simulink model "ev3_gyroboy_simulink_tcpip"  (R2024a)
settings: Solver=FixedStepDiscrete  StartTime=0.0  StopTime=inf  FixedStep=T_sampling  RelTol=1e-3  EnableMultiTasking=on
undefined symbols (not defined in the file): backward_speed, D_increment, D_max, D_min, DiscIntNeverNeededParam, forward_speed, initial_tilt, k_D_move, k_D_tilt, k_P_move, k_P_tilt, P_increment, P_max, P_min, T_sampling, tilt_limit, turning_speed
libraries: legoev3lib x19, powerlib_meascontrol x2, simulink x1, simulink_extras x1
settings Model: ExtModeTrigDuration=2  Creator=Barteq
settings SolverCC: AlgebraicLoopSolver=TrustRegion  PositivePriorityOrder=on
settings DataIOCC: ReturnWorkspaceOutputs=off
settings OptimizationCC: EnhancedBackFolding=on  PassReuseOutputArgsThreshold=0  MaxStackSize=64  OptimizeBlockOrder=speed  DifferentSizesBufferReuse=on  OptimizationCustomize=off
settings DebuggingCC: ParameterTunabilityLossMsg=error  UnconnectedInputMsg=warning  UnconnectedOutputMsg=warning  UnconnectedLineMsg=warning  ArithmeticOperatorsInVariantConditions=warning
settings HardwareCC: ProdBitPerPointer=32  ProdBitPerSizeT=32  ProdBitPerPtrDiffT=32  ProdLargestAtomicInteger=Long  ProdWordSize=32  ProdHWDeviceType=ARM Compatible->ARM 9
settings ModelReferenceCC: EnableRefExpFcnMdlSchedulingChecks=on
settings SFSimCC: SimUseLocalCustomCode=off  MATLABDynamicMemAlloc=off  CustomCodeUndefinedFunction=UseInterfaceOnly
settings RTWCC: Description=Embedded Coder  SystemTargetFile=ert.tlc  HardwareBoard=LEGO MINDSTORMS EV3  TLCOptions="-aInlineSetEventsForThisBaseRateFcn=TLC_FALSE -aSuppressMultiTaskScheduler=TLC_FALSE  -aRateBasedStepFcn=0"  TemplateMakefile=ert_default_tmf  RTWUseLocalCustomCode=off  Toolchain=Sourcery G++ Lite v2009q3  GPUComputeCapability=3.5
settings CodeAppCC: ForceParamTrailComments=on  OperatorAnnotations=on
settings ERTTargetCC: ERTCustomFileBanners=off  SupportContinuousTime=on  SupportNonInlinedSFcns=on  RemoveResetFunc=off  SupportVariableSizeSignals=on  ModelStepFunctionPrototypeControlCompliant=off
settings ConfigComp: CovBoundaryAbsTol=1.0e-5

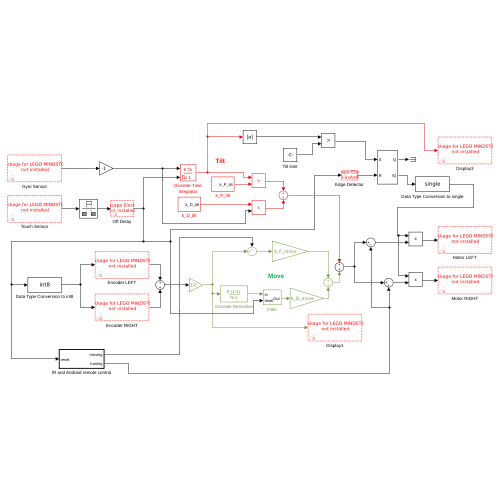
[thumbnail: Simulink's stored preview of the top-level diagram]
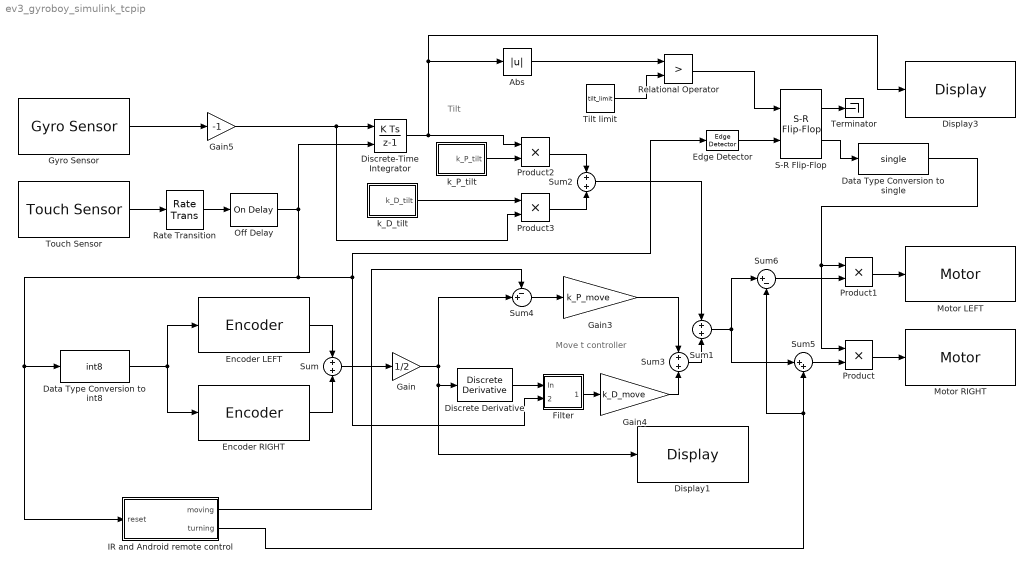
== system ev3_gyroboy_simulink_tcpip ==
  note: Tilt
  note: Move
      | t controller
  Abs : Abs  SaturateOnIntegerOverflow=off
  Data Type Conversion to int8 : DataTypeConversion  OutDataTypeStr=int8  SaturateOnIntegerOverflow=off  RndMeth=Floor
  Data Type Conversion to single : DataTypeConversion  OutDataTypeStr=single  SaturateOnIntegerOverflow=off  RndMeth=Floor
  Discrete Derivative : simulink/Discrete/Discrete Derivative  gainval=1.0  ICPrevScaledInput=0.0  OutMin=[]  OutMax=[]  OutDataTypeStr=single  OutputDataTypeScalingMode=single  OutDataType=fixdt(1, 16)  OutScaling=2^-10  DoSatur=off
  Discrete-Time Integrator : DiscreteIntegrator  ExternalReset=level  InitialCondition=initial_tilt  SampleTime=T_sampling  OutDataTypeStr=single  ICPrevOutput=DiscIntNeverNeededParam  ICPrevScaledInput=DiscIntNeverNeededParam
  Display1 : legoev3lib/Display  slcdStr=Encoders  slcdLine=6  slcdFormat=Decimal
      settings: SourceProductName=Simulink Support Package for LEGO MINDSTORMS EV3 Hardware
  Display3 : legoev3lib/Display  slcdStr=Tilt  slcdLine=4  slcdFormat=Decimal
      settings: SourceProductName=Simulink Support Package for LEGO MINDSTORMS EV3 Hardware
  Edge Detector : powerlib_meascontrol/Logic/Edge Detector  model=Falling  ic=0  Ts=T_sampling
      settings: SourceProductName=Simscape Power Systems
  Encoder LEFT : legoev3lib/Encoder  portNumber=B  opMode=Reset by external signal  sampleTime=T_sampling
      settings: SourceProductName=Simulink Support Package for LEGO MINDSTORMS EV3 Hardware
  Encoder RIGHT : legoev3lib/Encoder  portNumber=D  opMode=Reset by external signal  sampleTime=T_sampling
      settings: SourceProductName=Simulink Support Package for LEGO MINDSTORMS EV3 Hardware
  Filter : Subsystem
  Gain : Gain  Gain=1/2
  Gain3 : Gain  Gain=k_P_move
  Gain4 : Gain  Gain=k_D_move
  Gain5 : Gain  Gain=-1  OutDataTypeStr=single
  Gyro Sensor : legoev3lib/Gyro Sensor  portNumber=2  sampleTime=T_sampling
      settings: SourceProductName=Simulink Support Package for LEGO MINDSTORMS EV3 Hardware
  IR and Android remote control : Subsystem  TreatAsAtomicUnit=on
  Motor LEFT : legoev3lib/Motor  sportNumber=B  sstopAction=Brake
  Motor RIGHT : legoev3lib/Motor  sportNumber=D  sstopAction=Brake
  Off Delay : powerlib_meascontrol/Logic/On Delay  DelayType=Off delay  delay=delay_time  ic=1  Ts=T_sampling
      settings: SourceProductName=Simscape Power Systems
  Product{,1..3} (4 alike) : Product
  Rate Transition : RateTransition  OutPortSampleTime=T_sampling
  Relational Operator : RelationalOperator  Operator=>  OutDataTypeStr=boolean  RndMeth=Simplest  InputSameDT=off
  S-R Flip-Flop : simulink_extras/Flip Flops/S-R Flip-Flop  initial_condition=0
  Sum{,1..3} (4 alike) : Sum  OutDataTypeStr=single  AccumDataTypeStr=single
  Sum4 : Sum  Inputs=-+|  OutDataTypeStr=single  AccumDataTypeStr=single
  Sum5 : Sum  Inputs=|++  OutDataTypeStr=single  AccumDataTypeStr=single
  Sum6 : Sum  Inputs=|+-  OutDataTypeStr=single  AccumDataTypeStr=single
  Terminator : Terminator
  Tilt limit : Constant  Value=tilt_limit  OutDataTypeStr=single  SampleTime=T_sampling
  Touch Sensor : legoev3lib/Touch Sensor  portNumber=1  sampleTime=T_sampling*10
      settings: SourceProductName=Simulink Support Package for LEGO MINDSTORMS EV3 Hardware
  k_D_tilt : Subsystem
  k_P_tilt : Subsystem
  wires:
  Encoder LEFT/1 -> Sum/1
  Encoder RIGHT/1 -> Sum/2
  Sum/1 -> Gain/1
  Gain/1 -> Display1/1, Discrete Derivative/1, Sum4/2
  Filter/1(Out) -> Gain4/1
  Discrete-Time Integrator/1 -> Display3/1, Abs/1, Product2/1
  Gyro Sensor/1 -> Gain5/1
  Gain3/1 -> Sum3/1
  Gain4/1 -> Sum3/2
  Gain5/1 -> Product3/2, Discrete-Time Integrator/1
  Abs/1 -> Relational Operator/1
  Tilt limit/1 -> Relational Operator/2
  Relational Operator/1 -> S-R Flip-Flop/1
  Sum1/1 -> Sum6/1, Sum5/1
  S-R Flip-Flop/2 -> Data Type Conversion to single/1
  Touch Sensor/1 -> Rate Transition/1
  Data Type Conversion to int8/1 -> Encoder LEFT/1, Encoder RIGHT/1
  S-R Flip-Flop/1 -> Terminator/1
  Product2/1 -> Sum2/1
  Product3/1 -> Sum2/2
  Sum2/1 -> Sum1/1
  Sum3/1 -> Sum1/2
  Sum4/1 -> Gain3/1
  IR and Android remote control/2(turning) -> Sum6/2, Sum5/2
  IR and Android remote control/1(moving) -> Sum4/1
  Sum5/1 -> Product/2
  Product/1 -> Motor RIGHT/1
  Product1/1 -> Motor LEFT/1
  Sum6/1 -> Product1/2
  Data Type Conversion to single/1 -> Product/1, Product1/1
  k_P_tilt/1(k_P_tilt) -> Product2/2
  k_D_tilt/1(k_D_tilt) -> Product3/1
  Off Delay/1 -> IR and Android remote control/1(reset), Data Type Conversion to int8/1, Edge Detector/1, Filter/2(reset), Discrete-Time Integrator/2
  Rate Transition/1 -> Off Delay/1
  Edge Detector/1 -> S-R Flip-Flop/2
  Discrete Derivative/1 -> Filter/1(In)

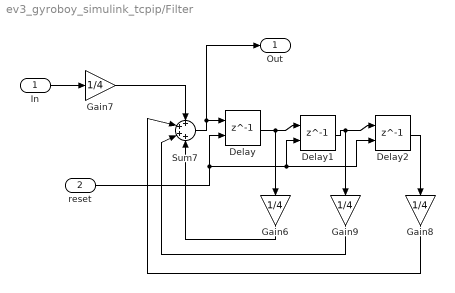
== system ev3_gyroboy_simulink_tcpip/Filter ==
  In : Inport
  reset : Inport  Port=2
  Delay : Delay  DelayLength=1  ExternalReset=Level  SampleTime=T_sampling
      settings: InputPortMap=u0,r5
  Delay1 : Delay  DelayLength=1  ExternalReset=Level  SampleTime=T_sampling
      settings: InputPortMap=u0,r5
  Delay2 : Delay  DelayLength=1  ExternalReset=Level  SampleTime=T_sampling
      settings: InputPortMap=u0,r5
  Gain{6..9} (4 alike) : Gain  Gain=1/4
  Sum7 : Sum  Inputs=++++  OutDataTypeStr=single  AccumDataTypeStr=single
  Out : Outport  VectorParamsAs1DForOutWhenUnconnected=off
  wires:
  Delay2/1 -> Gain8/1
  Gain8/1 -> Sum7/2
  In/1 -> Gain7/1
  Delay/1 -> Delay1/1, Gain6/1
  Sum7/1 -> Out/1, Delay/1
  Gain6/1 -> Sum7/4
  Delay1/1 -> Delay2/1, Gain9/1
  Gain7/1 -> Sum7/1
  Gain9/1 -> Sum7/3
  reset/1 -> Delay2/2, Delay1/2, Delay/2

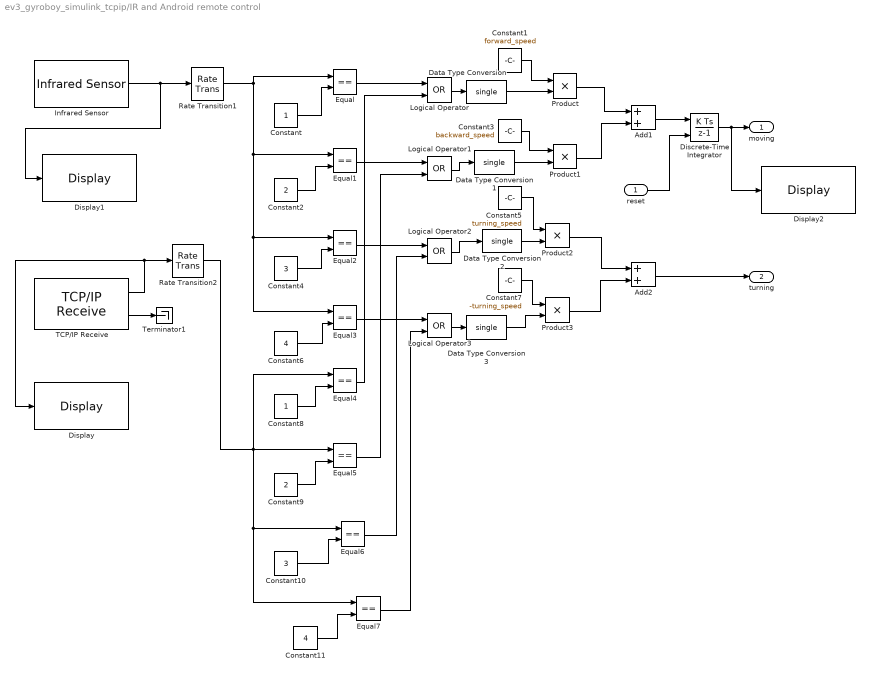
== system ev3_gyroboy_simulink_tcpip/IR and Android remote control ==
  reset : Inport
  Add1 : Sum
  Add2 : Sum
  Constant : Constant  SampleTime=T_sampling
  Constant1 : Constant  Value=forward_speed  OutDataTypeStr=single  SampleTime=T_sampling
  Constant10 : Constant  Value=3  SampleTime=T_sampling
  Constant11 : Constant  Value=4  SampleTime=T_sampling
  Constant2 : Constant  Value=2  SampleTime=T_sampling
  Constant3 : Constant  Value=backward_speed  OutDataTypeStr=single  SampleTime=T_sampling
  Constant4 : Constant  Value=3  SampleTime=T_sampling
  Constant5 : Constant  Value=turning_speed  OutDataTypeStr=single  SampleTime=T_sampling
  Constant6 : Constant  Value=4  SampleTime=T_sampling
  Constant7 : Constant  Value=-turning_speed  OutDataTypeStr=single  SampleTime=T_sampling
  Constant8 : Constant  SampleTime=T_sampling
  Constant9 : Constant  Value=2  SampleTime=T_sampling
  Data Type Conversion{,1..3} (4 alike) : DataTypeConversion  OutDataTypeStr=single  SaturateOnIntegerOverflow=off  RndMeth=Floor
  Discrete-Time Integrator : DiscreteIntegrator  ExternalReset=level  SampleTime=T_sampling  ICPrevOutput=DiscIntNeverNeededParam  ICPrevScaledInput=DiscIntNeverNeededParam
  Display : legoev3lib/Display  slcdStr=Android  slcdLine=1  slcdFormat=Decimal
      settings: SourceProductName=Simulink Support Package for LEGO MINDSTORMS EV3 Hardware
  Display1 : legoev3lib/Display  slcdStr=Remote  slcdLine=2  slcdFormat=Decimal
      settings: SourceProductName=Simulink Support Package for LEGO MINDSTORMS EV3 Hardware
  Display2 : legoev3lib/Display  slcdStr=Moving  slcdLine=3  slcdFormat=Decimal
      settings: SourceProductName=Simulink Support Package for LEGO MINDSTORMS EV3 Hardware
  Equal{,1..7} (8 alike) : RelationalOperator  Operator===  OutDataTypeStr=boolean  RndMeth=Simplest  InputSameDT=off
  Infrared Sensor : legoev3lib/Infrared Sensor  Parameter5=on  portNumber=4  mode=Remote  channel=1  SampleTime=T_sampling*10
      settings: SourceProductName=Simulink Support Package for LEGO MINDSTORMS EV3 Hardware
  Logical Operator{,1..3} (4 alike) : Logic  Operator=OR  AllPortsSameDT=off  OutDataTypeStr=boolean
  Product{,1..3} (4 alike) : Product
  Rate Transition1 : RateTransition  OutPortSampleTime=T_sampling
  Rate Transition2 : RateTransition  OutPortSampleTime=T_sampling
  TCP/IP Receive : legoev3lib/TCP//IP Receive  Mode_=Server  LocalServerPort_=25000  RemoteAddr_=127.0.0.1  RemoteServerPort_=25000  DataType_=int8  DataSize_=1  SampleTime_=T_sampling*10  SimulateUsing=Code generation  ClientPortBindingSelection_=off  ClientPortToBind_=35000  BlockingMode_=off  BlockTimeout_=0.1
      settings: SourceProductName=Simulink Support Package for LEGO MINDSTORMS EV3 Hardware
  Terminator1 : Terminator
  moving : Outport  VectorParamsAs1DForOutWhenUnconnected=off
  turning : Outport  Port=2  VectorParamsAs1DForOutWhenUnconnected=off
  wires:
  Discrete-Time Integrator/1 -> Display2/1, moving/1
  Constant/1 -> Equal/2
  Product/1 -> Add1/1
  Constant1/1 -> Product/1
  Data Type Conversion/1 -> Product/2
  Data Type Conversion1/1 -> Product1/2
  Constant2/1 -> Equal1/2
  Constant3/1 -> Product1/1
  Product1/1 -> Add1/2
  Add1/1 -> Discrete-Time Integrator/1
  Constant4/1 -> Equal2/2
  Constant7/1 -> Product3/1
  Constant6/1 -> Equal3/2
  Data Type Conversion2/1 -> Product2/2
  Constant5/1 -> Product2/1
  Product2/1 -> Add2/1
  Infrared Sensor/1 -> Display1/1, Rate Transition1/1
  Data Type Conversion3/1 -> Product3/2
  Product3/1 -> Add2/2
  Add2/1 -> turning/1
  reset/1 -> Discrete-Time Integrator/2
  TCP/IP Receive/2 -> Terminator1/1
  Constant11/1 -> Equal7/2
  Constant10/1 -> Equal6/2
  Constant9/1 -> Equal5/2
  Constant8/1 -> Equal4/2
  Logical Operator/1 -> Data Type Conversion/1
  Equal/1 -> Logical Operator/1
  Equal4/1 -> Logical Operator/2
  Equal1/1 -> Logical Operator1/1
  Logical Operator1/1 -> Data Type Conversion1/1
  Equal5/1 -> Logical Operator1/2
  Logical Operator2/1 -> Data Type Conversion2/1
  Equal2/1 -> Logical Operator2/1
  Equal6/1 -> Logical Operator2/2
  Logical Operator3/1 -> Data Type Conversion3/1
  Equal3/1 -> Logical Operator3/1
  Equal7/1 -> Logical Operator3/2
  TCP/IP Receive/1 -> Rate Transition2/1, Display/1
  Rate Transition1/1 -> Equal/1, Equal3/1, Equal2/1, Equal1/1
  Rate Transition2/1 -> Equal4/1, Equal7/1, Equal6/1, Equal5/1

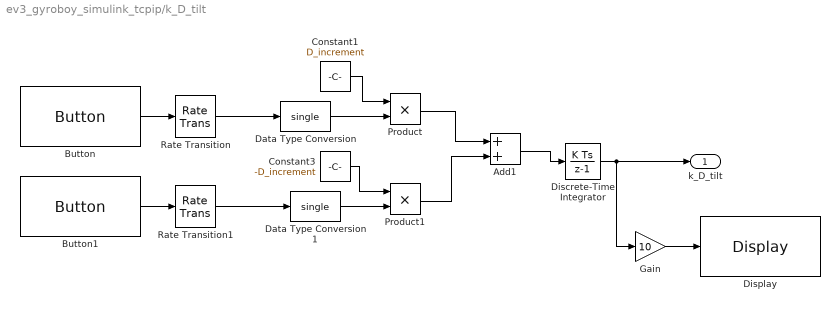
== system ev3_gyroboy_simulink_tcpip/k_D_tilt ==
  Add1 : Sum
  Button : legoev3lib/Button  buttonType=Right  sampleTime=T_sampling
      settings: SourceProductName=Simulink Support Package for LEGO MINDSTORMS EV3 Hardware
  Button1 : legoev3lib/Button  buttonType=Left  sampleTime=T_sampling
      settings: SourceProductName=Simulink Support Package for LEGO MINDSTORMS EV3 Hardware
  Constant1 : Constant  Value=D_increment  OutDataTypeStr=single  SampleTime=T_sampling
  Constant3 : Constant  Value=-D_increment  OutDataTypeStr=single  SampleTime=T_sampling
  Data Type Conversion : DataTypeConversion  OutDataTypeStr=single  SaturateOnIntegerOverflow=off  RndMeth=Floor
  Data Type Conversion1 : DataTypeConversion  OutDataTypeStr=single  SaturateOnIntegerOverflow=off  RndMeth=Floor
  Discrete-Time Integrator : DiscreteIntegrator  InitialCondition=k_D_tilt  SampleTime=T_sampling  LimitOutput=on  UpperSaturationLimit=D_max  LowerSaturationLimit=D_min  ICPrevOutput=DiscIntNeverNeededParam  ICPrevScaledInput=DiscIntNeverNeededParam
  Display : legoev3lib/Display  slcdStr=k_D_10x  slcdLine=10  slcdFormat=Decimal
      settings: SourceProductName=Simulink Support Package for LEGO MINDSTORMS EV3 Hardware
  Gain : Gain  Gain=10
  Product : Product
  Product1 : Product
  Rate Transition : RateTransition  OutPortSampleTime=T_sampling
  Rate Transition1 : RateTransition  OutPortSampleTime=T_sampling
  k_D_tilt : Outport  VectorParamsAs1DForOutWhenUnconnected=off
  wires:
  Rate Transition1/1 -> Data Type Conversion1/1
  Add1/1 -> Discrete-Time Integrator/1
  Rate Transition/1 -> Data Type Conversion/1
  Product/1 -> Add1/1
  Data Type Conversion/1 -> Product/2
  Discrete-Time Integrator/1 -> Gain/1, k_D_tilt/1
  Product1/1 -> Add1/2
  Constant1/1 -> Product/1
  Data Type Conversion1/1 -> Product1/2
  Constant3/1 -> Product1/1
  Button/1 -> Rate Transition/1
  Button1/1 -> Rate Transition1/1
  Gain/1 -> Display/1

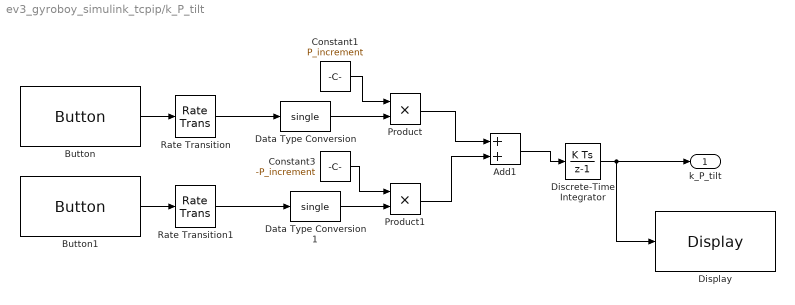
== system ev3_gyroboy_simulink_tcpip/k_P_tilt ==
  Add1 : Sum
  Button : legoev3lib/Button  buttonType=Up  sampleTime=T_sampling
      settings: SourceProductName=Simulink Support Package for LEGO MINDSTORMS EV3 Hardware
  Button1 : legoev3lib/Button  buttonType=Down  sampleTime=T_sampling
      settings: SourceProductName=Simulink Support Package for LEGO MINDSTORMS EV3 Hardware
  Constant1 : Constant  Value=P_increment  OutDataTypeStr=single  SampleTime=T_sampling
  Constant3 : Constant  Value=-P_increment  OutDataTypeStr=single  SampleTime=T_sampling
  Data Type Conversion : DataTypeConversion  OutDataTypeStr=single  SaturateOnIntegerOverflow=off  RndMeth=Floor
  Data Type Conversion1 : DataTypeConversion  OutDataTypeStr=single  SaturateOnIntegerOverflow=off  RndMeth=Floor
  Discrete-Time Integrator : DiscreteIntegrator  InitialCondition=k_P_tilt  SampleTime=T_sampling  LimitOutput=on  UpperSaturationLimit=P_max  LowerSaturationLimit=P_min  ICPrevOutput=DiscIntNeverNeededParam  ICPrevScaledInput=DiscIntNeverNeededParam
  Display : legoev3lib/Display  slcdStr=k_P_tilt  slcdLine=9  slcdFormat=Decimal
      settings: SourceProductName=Simulink Support Package for LEGO MINDSTORMS EV3 Hardware
  Product : Product
  Product1 : Product
  Rate Transition : RateTransition  OutPortSampleTime=T_sampling
  Rate Transition1 : RateTransition  OutPortSampleTime=T_sampling
  k_P_tilt : Outport  VectorParamsAs1DForOutWhenUnconnected=off
  wires:
  Rate Transition1/1 -> Data Type Conversion1/1
  Add1/1 -> Discrete-Time Integrator/1
  Rate Transition/1 -> Data Type Conversion/1
  Product/1 -> Add1/1
  Data Type Conversion/1 -> Product/2
  Discrete-Time Integrator/1 -> Display/1, k_P_tilt/1
  Product1/1 -> Add1/2
  Constant1/1 -> Product/1
  Data Type Conversion1/1 -> Product1/2
  Constant3/1 -> Product1/1
  Button/1 -> Rate Transition/1
  Button1/1 -> Rate Transition1/1
